simulink model "untitled"  (R2021a)
settings: Solver=ode15s  StartTime=0.0  StopTime=10.0  RelTol=1e-3
settings Model: Creator=MikeyG  LastModifiedBy=MikeyG
settings SolverCC: MaxConsecutiveMinStep=2  AlgebraicLoopSolver=TrustRegion
settings DataIOCC: SaveFormat=Array
settings DebuggingCC: SFMachineParentedDataDiag=warning

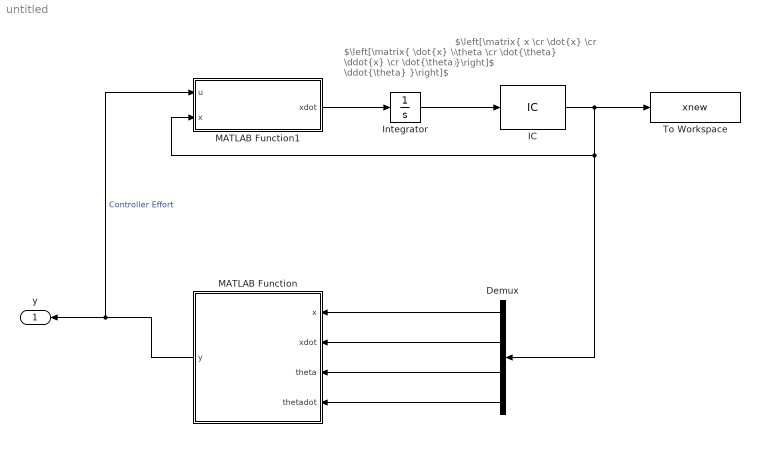
== system untitled ==
  note: $\left[\matrix{ \dot{x} \cr \ddot{x} \cr \dot{\theta} \cr \ddot{\theta} }\right]$
  note: $\left[\matrix{ x \cr \dot{x} \cr \theta \cr \dot{\theta} }\right]$
  Demux : Demux
  IC : InitialCondition  Value=[0;0;pi/10;0]
  Integrator : Integrator
  MATLAB Function : MATLAB Function  TreatAsAtomicUnit=on
  MATLAB Function1 : MATLAB Function  TreatAsAtomicUnit=on
  To Workspace : ToWorkspace  VariableName=xnew  SaveFormat=Timeseries  SampleTime=-1
  y : Outport
  wires:
  MATLAB Function/1(y) -> MATLAB Function1/1(u), y/1  "Controller Effort"
  MATLAB Function1/1(xdot) -> Integrator/1
  Demux/1 -> MATLAB Function/1(x)
  Demux/2 -> MATLAB Function/2(xdot)
  Demux/4 -> MATLAB Function/4(thetadot)
  Integrator/1 -> IC/1
  Demux/3 -> MATLAB Function/3(theta)
  IC/1 -> To Workspace/1, MATLAB Function1/2(x), Demux/1

== matlab function untitled/MATLAB Function1 ==
  data: u input; x input; xdot output
function xdot  = fcn(u, x)

%     M = 10;
%     m = 2;
%     L = 0.66;
%     g = 9.8;
%     
%     % Deadzone
%     if (u < 0.1) && (u > -0.1)
%         u = 0;
%     end
%     
%     xdot = zeros(4,1);
%     
%     xdot(1,1) = x(2,1);
%     xdot(2,1) = (u+m*sin(x(3,1))*(L*x(4,1)^2-g*cos(x(3,1))))/ ...
%         (M+m*sin(x(3,1))^2);
%     xdot(3,1) = x(4,1);
%     xdot(4,1) = (-u*cos(x(3,1))-m*L*x(4,1)^2*sin(x(3,1))*cos(x(3,1))+(M+m)*g*sin(x(3,1)))/ ...
%         (L*(M+m*sin(x(3,1))^2));

    M = 10;
    m = 2;
    L = 0.66;
    g = 9.8;
    
    % Deadzone
    if (u < 0.1) && (u > -0.1)
        u = 0;
    end
    
    xdot = zeros(4,1);
    xdot(1,1) = x(2,1);
    xdot(2,1) = (u+m*sin(x(3,1))*(L*x(4,1)^2-g*cos(x(3,1))))/ ...
        (M+m*sin(x(3,1))^2);
    xdot(3,1) = x(4,1);
    xdot(4,1) = (-u*cos(x(3,1))-m*L*x(4,1)^2*sin(x(3,1))*cos(x(3,1))+(M+m)*g*sin(x(3,1)))/ ...
        (L*(M+m*sin(x(3,1))^2));

end

== matlab function untitled/MATLAB Function ==
  data: x input; y output; xdot input; theta input; thetadot input
function y = fcn(x, xdot, theta, thetadot)

y = simFunct(x,xdot,theta,thetadot);
